simulink model "CruiseControl_PI_Controller_Faiyaz_Edit_1"  (R2020a)
settings: Solver=ode45  StartTime=0.0  StopTime=40  RelTol=1e-3  AbsTol=1e-6
settings Model: Creator=Rick  LastModifiedBy=ashra
settings SolverCC: AutoScaleAbsTol=off
settings DataIOCC: SaveFormat=Array  SignalLoggingSaveFormat=ModelDataLogs  ReturnWorkspaceOutputs=off
settings OptimizationCC: BlockReduction=off  BooleanDataType=off  ExpressionDepthLimit=2147483647  LifeSpan=inf
settings DebuggingCC: SaveWithParameterizedLinksMsg=none  UnderspecifiedInitializationDetection=Classic  MergeDetectMultiDrivingBlocksExec=none  SignalResolutionControl=TryResolveAllWithWarning  MultiTaskDSMMsg=warning  MultiTaskCondExecSysMsg=none  FcnCallInpInsideContextMsg=warning  StateNameClashWarn=warning  SFUnexpectedBacktrackingDiag=warning  SFNoUnconditionalDefaultTransitionDiag=warning  SFExecutionAtInitializationDiag=none  ArithmeticOperatorsInVariantConditions=warning
settings HardwareCC: ProdBitPerPointer=32  ProdBitPerSizeT=32  ProdBitPerPtrDiffT=32  ProdLargestAtomicFloat=None  ProdIntDivRoundTo=Undefined  ProdEndianess=Unspecified  ProdWordSize=32  ProdHWDeviceType=32-bit Generic  TargetUnknown=on
settings ModelReferenceCC: PropagateSignalLabelsOutOfModel=off
settings SFSimCC: SimUseLocalCustomCode=off  CustomCodeUndefinedFunction=UseInterfaceOnly
settings RTWCC: RTWUseLocalCustomCode=off
settings CodeAppCC: StateflowObjectComments=on
settings GRTTargetCC: TargetLangStandard=C89/C90 (ANSI)
settings ConfigComp: CovMetricSettings=dw  CovHtmlReporting=on  CovSaveCumulativeToWorkspaceVar=on  CovSaveSingleToWorkspaceVar=on  CovExternalEMLEnable=off

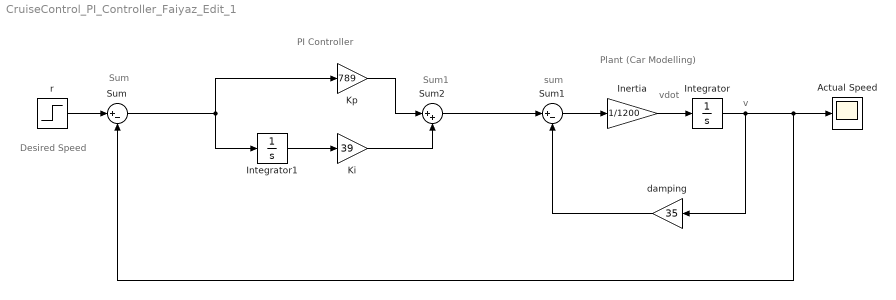
== system CruiseControl_PI_Controller_Faiyaz_Edit_1 ==
  note: PI Controller
  note: Desired Speed
  note: Plant (Car Modelling)
  note: Sum
  note: sum
  note: v
  note: vdot
  note: Sum1
  Actual Speed : Scope
  Inertia : Gain  Gain=1/1200
  Integrator : Integrator
  Integrator1 : Integrator
  Ki : Gain  Gain=39
  Kp : Gain  Gain=789
  Sum : Sum  Inputs=|+-
  Sum1 : Sum  Inputs=|+-
  Sum2 : Sum  Inputs=|++
  damping : Gain  Gain=35
  r : Step  Time=0  After=30
  wires:
  r/1 -> Sum/1
  Inertia/1 -> Integrator/1
  Sum1/1 -> Inertia/1
  damping/1 -> Sum1/2
  Integrator/1 -> Actual Speed/1, Sum/2, damping/1
  Ki/1 -> Sum2/2
  Integrator1/1 -> Ki/1
  Kp/1 -> Sum2/1
  Sum2/1 -> Sum1/1
  Sum/1 -> Integrator1/1, Kp/1
